simulink model "airspeedController"  (R2019a)
settings: Solver=VariableStepAuto  StartTime=0.0  StopTime=10.0  RelTol=1e-3
values from neighbouring files (symbols this model uses):
  D = diag([0 k1*k3 k4/d])    [airspeedController.m]    (also in forces_moments.m; forces_moments_testing.m; precisionLanding.m)
  g = 9.8    [airspeedController.m]    (also in precisionLanding.m = P.gravity)
  gama = 1    [airspeedController.m]    (also in forces_moments.m; forces_moments_testing.m; precisionLanding.m)
  k_VI = 0.8    [airspeedController.m]    (also in forces_moments.m; forces_moments_testing.m; main_precision_landing.m; precisionLanding.m)
  k_VP = 0.5    [airspeedController.m]    (also in forces_moments.m; forces_moments_testing.m; main_precision_landing.m; precisionLanding.m)
  mass = 25    [airspeedController.m]    (also in precisionLanding.m = P.mass)
settings Model: Creator=gcmsm  LastModifiedBy=gcmsm

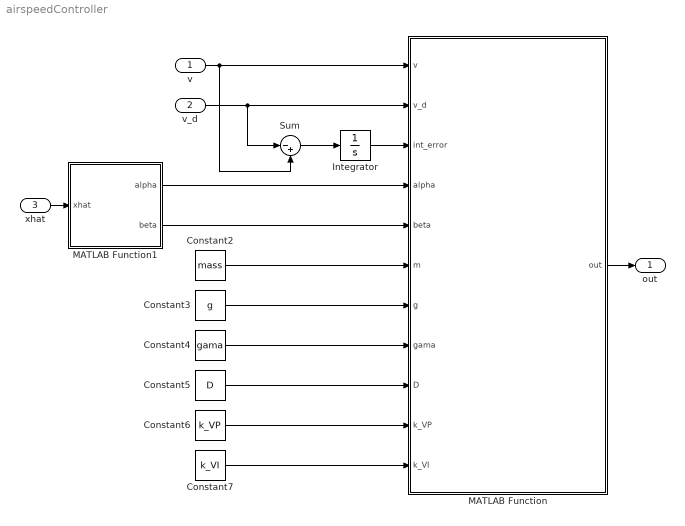
== system airspeedController ==
  "v " : Inport
  v_d : Inport  Port=2
  xhat : Inport  Port=3
  Constant2 : Constant  Value=mass
  Constant3 : Constant  Value=g
  Constant4 : Constant  Value=gama
  Constant5 : Constant  Value=D
  Constant6 : Constant  Value=k_VP
  Constant7 : Constant  Value=k_VI
  Integrator : Integrator
  MATLAB Function : MATLAB Function  TreatAsAtomicUnit=on
  MATLAB Function1 : MATLAB Function  TreatAsAtomicUnit=on
  Sum : Sum  Inputs=|-+
  "out " : Outport
  wires:
  "v "/1 -> Sum/2, MATLAB Function/1(v)
  Sum/1 -> Integrator/1
  v_d/1 -> Sum/1, MATLAB Function/2(v_d)
  Integrator/1 -> MATLAB Function/3(int_error)
  MATLAB Function1/1(alpha) -> MATLAB Function/4(alpha)
  MATLAB Function1/2(beta) -> MATLAB Function/5(beta)
  Constant2/1 -> MATLAB Function/6(m)
  Constant3/1 -> MATLAB Function/7(g)
  Constant4/1 -> MATLAB Function/8(gama)
  Constant5/1 -> MATLAB Function/9(D)
  Constant6/1 -> MATLAB Function/10(k_VP)
  Constant7/1 -> MATLAB Function/11(k_VI)
  MATLAB Function/1(out) -> "out "/1
  xhat/1 -> MATLAB Function1/1(xhat)

== matlab function airspeedController/MATLAB Function1 ==
  data: alpha output; xhat input; beta output
function [alpha,beta] = getData(xhat)
    alpha = xhat(5);
    beta = xhat(6);
end

== matlab function airspeedController/MATLAB Function ==
  data: v input; v_d input; out output; int_error input; alpha input; beta input; m input; g input; gama input; D input; k_VP input; k_VI input
function out = airspeedController(v,v_d,int_error,alpha,beta,m,g,gama,D,k_VP,k_VI)


F_T = [(D + mass*g*sin(gama)/(cos(beta)*cos(alpha))] + ...
      [(k_VP*(v-v_d) + k_VI*int_error)/(cos(beta)*cos(alpha))];

end
